simulink model "analisisDinamico2017"  (R2017a)
settings: Solver=VariableStepAuto  StartTime=0.0  StopTime=fin  FixedStep=0.001  RelTol=1e-3
values from neighbouring files (symbols this model uses):
  Aa1 = 1    [A_1_Obtencion_Modelo_Simbolico.m]    (also in modeloSimbolico.mat)
  Aa2 = Im2_cc*0.7    (= 2.59)    [A_1_Obtencion_Modelo_Simbolico.m]    (also in modeloSimbolico.mat)
  Aa3 = Im3_cc*0.6    (= 0.6)    [A_1_Obtencion_Modelo_Simbolico.m]    (also in modeloSimbolico.mat)
  Ab1 = 0.5    [A_1_Obtencion_Modelo_Simbolico.m]    (also in modeloSimbolico.mat)
  Ab2 = Aa2*0.8    (= 2.072)    [A_1_Obtencion_Modelo_Simbolico.m]    (also in modeloSimbolico.mat)
  Ab3 = Aa3*0.62    (= 0.372)    [A_1_Obtencion_Modelo_Simbolico.m]    (also in modeloSimbolico.mat)
  noise = 0.01    [A_1_Obtencion_Modelo_Simbolico.m]    (also in modeloSimbolico.mat)
  q2ini = -0.80020550259323    (= -0.800205502593)    [A_1_Obtencion_Modelo_Simbolico.m]    (also in modeloSimbolico.mat)
  q3ini = 0.202600802956157    (= 0.202600802956)    [A_1_Obtencion_Modelo_Simbolico.m]    (also in modeloSimbolico.mat)
  R1 = 50    [A_1_Obtencion_Modelo_Simbolico.m]    (also in A_2_Modelo_medidas_muestreado.m; A_2_Modelo_medidas_perfectas.m; modeloSimbolico.mat)
  R2 = 30    [A_1_Obtencion_Modelo_Simbolico.m]    (also in A_2_Modelo_medidas_muestreado.m; A_2_Modelo_medidas_perfectas.m; modeloSimbolico.mat)
  R3 = 15    [A_1_Obtencion_Modelo_Simbolico.m]    (also in A_2_Modelo_medidas_muestreado.m; A_2_Modelo_medidas_perfectas.m; modeloSimbolico.mat)
  Tau1 = 8    [A_1_Obtencion_Modelo_Simbolico.m]    (also in modeloSimbolico.mat)
  Tau2 = 15    [A_1_Obtencion_Modelo_Simbolico.m]    (also in modeloSimbolico.mat)
  Tau3 = 20    [A_1_Obtencion_Modelo_Simbolico.m]    (also in modeloSimbolico.mat)
  Ts = 0.001    [A_1_Obtencion_Modelo_Simbolico.m]    (also in modeloSimbolico.mat)
  wa1 = 1.3    [A_1_Obtencion_Modelo_Simbolico.m]    (also in modeloSimbolico.mat)
  wa2 = 3    [A_1_Obtencion_Modelo_Simbolico.m]    (also in modeloSimbolico.mat)
  wa3 = 5    [A_1_Obtencion_Modelo_Simbolico.m]    (also in modeloSimbolico.mat)
  wb1 = wa1*5    (= 6.5)    [A_1_Obtencion_Modelo_Simbolico.m]    (also in modeloSimbolico.mat)
  wb2 = wa2*3.5    (= 10.5)    [A_1_Obtencion_Modelo_Simbolico.m]    (also in modeloSimbolico.mat)
  wb3 = wa3*2.2    (= 11)    [A_1_Obtencion_Modelo_Simbolico.m]    (also in modeloSimbolico.mat)
undefined symbols (not defined in the file or in its folder): modeloIdeal, modeloReal
settings Model: Creator=Richa  LastModifiedBy=richard

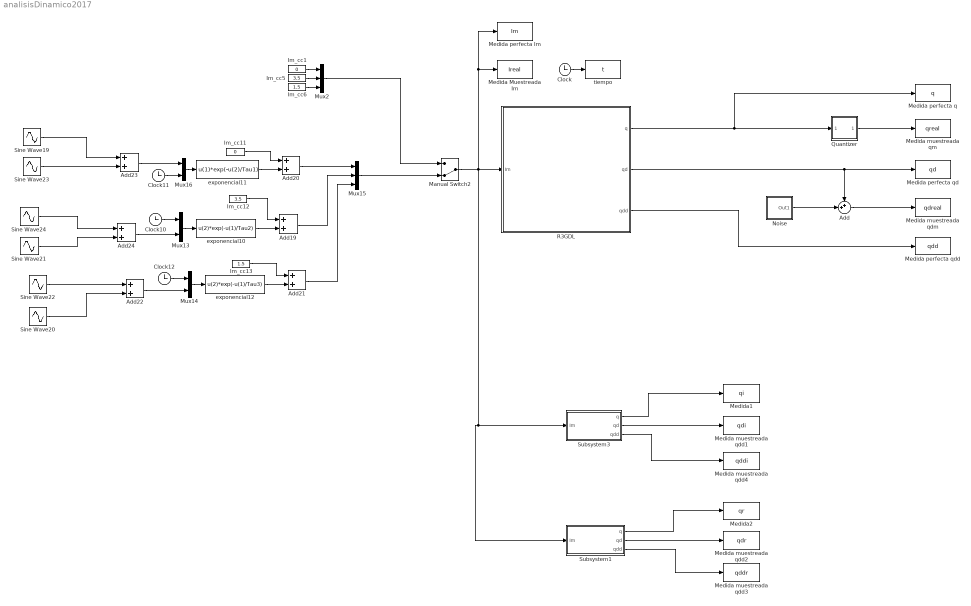
== system analisisDinamico2017 ==
  Add : Sum  Inputs=++|
  Add{19..24} (6 alike) : Sum
  Clock{,10..12} (4 alike) : Clock
  Im_cc1 : Constant  Value=0
  Im_cc11 : Constant  Value=0
  Im_cc12 : Constant  Value=3.5
  Im_cc13 : Constant  Value=1.5
  Im_cc5 : Constant  Value=3.5
  Im_cc6 : Constant  Value=1.5
  Manual Switch2 : ManualSwitch  CurrentSetting=0
  Medida Muestreada Im : ToWorkspace  VariableName=Ireal  SampleTime=Ts
  Medida muestreada qdd1 : ToWorkspace  VariableName=qdi  SampleTime=Ts
  Medida muestreada qdd2 : ToWorkspace  VariableName=qdr  SampleTime=Ts
  Medida muestreada qdd3 : ToWorkspace  VariableName=qddr  SampleTime=Ts
  Medida muestreada qdd4 : ToWorkspace  VariableName=qddi  SampleTime=Ts
  Medida muestreada qdm : ToWorkspace  VariableName=qdreal  SampleTime=Ts
  Medida muestreada qm : ToWorkspace  VariableName=qreal  SampleTime=Ts
  Medida perfecta Im : ToWorkspace  VariableName=Im  SampleTime=-1
  Medida perfecta q : ToWorkspace  VariableName=q  SampleTime=-1
  Medida perfecta qd : ToWorkspace  VariableName=qd  SampleTime=-1
  Medida perfecta qdd : ToWorkspace  VariableName=qdd  SampleTime=-1
  Medida1 : ToWorkspace  VariableName=qi  SampleTime=Ts
  Medida2 : ToWorkspace  VariableName=qr  SampleTime=Ts
  Mux13 : Mux  Inputs=2
  Mux14 : Mux  Inputs=2
  Mux15 : Mux  Inputs=3
  Mux16 : Mux  Inputs=2
  Mux2 : Mux  Inputs=3
  "Noise " : Subsystem
  "Quantizer " : Subsystem
  R3GDL : Subsystem  mask(Control y Programación de Robots (4 GIERM)){NGrupo=15, q1_ini=0, q2_ini=q2ini, q3_ini=q3ini, Bl_q1=off, Bl_q2=off, Bl_q3=off, AccionamientoDirecto=off}
      mask prompts: NGrupo "Nº de GRUPO"; q1_ini "q1 inicial  (rad)"; q2_ini "q2 inicial (rad)"; q3_ini "q3_inicial (rad)"; Bl_q1 "Bloqueo q1"; Bl_q2 "Bloqueo q2"; Bl_q3 "Bloqueo q3"; AccionamientoDirecto "Accionamiento directo"
      mask help: Robot de 3 grados de libertad RRR
      mask Display:
      | image(imread('R3GDL_RRR.JPG'));
      | port_label('output', 1, 'q');
      | port_label('output', 2, 'qd');
      | port_label('output', 3, 'qdd');
      | port_label('input', 1, 'Im')
  Sine Wave19 : Sin  Amplitude=Aa1  Frequency=wa1  SampleTime=0
  Sine Wave20 : Sin  Amplitude=Ab3  Frequency=wb3  SampleTime=0
  Sine Wave21 : Sin  Amplitude=Ab2  Frequency=wb2  SampleTime=0
  Sine Wave22 : Sin  Amplitude=Aa3  Frequency=wa3  SampleTime=0
  Sine Wave23 : Sin  Amplitude=Ab1  Frequency=wb1  SampleTime=0
  Sine Wave24 : Sin  Amplitude=Aa2  Frequency=wa2  SampleTime=0
  Subsystem1 : Subsystem
  Subsystem3 : Subsystem
  exponencial10 : Fcn  Expr=u(2)*exp(-u(1)/Tau2)
  exponencial11 : Fcn  Expr=u(1)*exp(-u(2)/Tau1)
  exponencial12 : Fcn  Expr=u(2)*exp(-u(1)/Tau3)
  tiempo : ToWorkspace  VariableName=t  SampleTime=Ts
  wires:
  "Quantizer "/1(Out1) -> Medida muestreada qm/1
  R3GDL/1(q) -> Medida perfecta q/1, "Quantizer "/1(In1)
  R3GDL/2(qd) -> Medida perfecta qd/1, Add/1
  "Noise "/1(Out1) -> Add/2
  Add/1 -> Medida muestreada qdm/1
  R3GDL/3(qdd) -> Medida perfecta qdd/1
  Manual Switch2/1 -> Medida perfecta Im/1, Medida Muestreada Im/1, Subsystem1/1(Im), Subsystem3/1(Im), R3GDL/1(Im)
  Clock/1 -> tiempo/1
  Add19/1 -> Mux15/2
  Im_cc12/1 -> Add19/1
  Clock10/1 -> Mux13/1
  Mux13/1 -> exponencial10/1
  exponencial10/1 -> Add19/2
  Add24/1 -> Mux13/2
  Sine Wave24/1 -> Add24/1
  Sine Wave21/1 -> Add24/2
  Add21/1 -> Mux15/3
  Mux14/1 -> exponencial12/1
  Clock12/1 -> Mux14/1
  Sine Wave20/1 -> Add22/2
  Add22/1 -> Mux14/2
  exponencial12/1 -> Add21/2
  Sine Wave22/1 -> Add22/1
  Im_cc13/1 -> Add21/1
  Im_cc11/1 -> Add20/1
  Clock11/1 -> Mux16/2
  Add23/1 -> Mux16/1
  Add20/1 -> Mux15/1
  Sine Wave23/1 -> Add23/2
  Mux16/1 -> exponencial11/1
  Sine Wave19/1 -> Add23/1
  exponencial11/1 -> Add20/2
  Mux2/1 -> Manual Switch2/1
  Im_cc1/1 -> Mux2/1
  Im_cc5/1 -> Mux2/2
  Im_cc6/1 -> Mux2/3
  Subsystem3/3(qdd) -> Medida muestreada qdd4/1
  Subsystem3/2(qd) -> Medida muestreada qdd1/1
  Subsystem3/1(q) -> Medida1/1
  Mux15/1 -> Manual Switch2/2
  Subsystem1/1(q) -> Medida2/1
  Subsystem1/2(qd) -> Medida muestreada qdd2/1
  Subsystem1/3(qdd) -> Medida muestreada qdd3/1

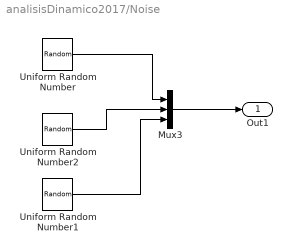
== system analisisDinamico2017/Noise  ==
  Mux3 : Mux  Inputs=3
  Uniform Random Number : UniformRandomNumber  Minimum=-(1500*2*pi/60)*(noise/R1)  Maximum=(1500*2*pi/60)*(noise/R1)  SampleTime=Ts*2
  Uniform Random Number1 : UniformRandomNumber  Minimum=-(1500*2*pi/60)*(noise/R3)  Maximum=(1500*2*pi/60)*(noise/R3)  SampleTime=Ts*2
  Uniform Random Number2 : UniformRandomNumber  Minimum=-(1500*2*pi/60)*(noise/R2)  Maximum=(1500*2*pi/60)*(noise/R2)  SampleTime=Ts*2
  Out1 : Outport
  wires:
  Uniform Random Number1/1 -> Mux3/3
  Uniform Random Number/1 -> Mux3/1
  Uniform Random Number2/1 -> Mux3/2
  Mux3/1 -> Out1/1

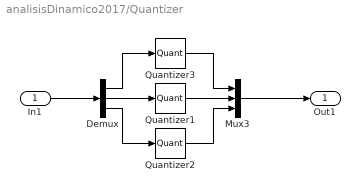
== system analisisDinamico2017/Quantizer  ==
  In1 : Inport
  Demux : Demux  Outputs=3
  Mux3 : Mux  Inputs=3
  Quantizer1 : Quantizer  QuantizationInterval=2*pi/1024/30
  Quantizer2 : Quantizer  QuantizationInterval=2*pi/1024/15
  Quantizer3 : Quantizer  QuantizationInterval=2*pi/1024/50
  Out1 : Outport
  wires:
  Demux/2 -> Quantizer1/1
  Mux3/1 -> Out1/1
  Quantizer1/1 -> Mux3/2
  Quantizer3/1 -> Mux3/1
  Quantizer2/1 -> Mux3/3
  In1/1 -> Demux/1
  Demux/3 -> Quantizer2/1
  Demux/1 -> Quantizer3/1

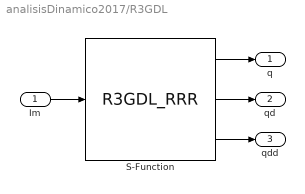
== system analisisDinamico2017/R3GDL ==
  Im : Inport
  S-Function : S-Function  FunctionName=R3GDL_RRR  Parameters=[q1_ini; q2_ini; q3_ini]; [Bl_q1; Bl_q2; Bl_q3]; AccionamientoDirecto; NGrupo  SFunctionDeploymentMode=off  EnableBusSupport=off
  q : Outport
  qd : Outport  Port=2
  qdd : Outport  Port=3
  wires:
  Im/1 -> S-Function/1
  S-Function/1 -> q/1
  S-Function/2 -> qd/1
  S-Function/3 -> qdd/1

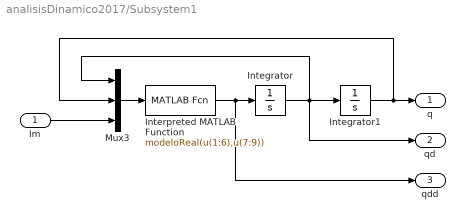
== system analisisDinamico2017/Subsystem1 ==
  Im : Inport
  Integrator : Integrator
  Integrator1 : Integrator  InitialCondition=[0 q2ini q3ini]
  Interpreted MATLAB Function : MATLABFcn  MATLABFcn=modeloReal(u(1:6),u(7:9))  OutputDimensions=3
  Mux3 : Mux  Inputs=3
  q : Outport
  qd : Outport  Port=2
  qdd : Outport  Port=3
  wires:
  Im/1 -> Mux3/3
  Integrator/1 -> Integrator1/1, Mux3/1, qd/1
  Interpreted MATLAB Function/1 -> qdd/1, Integrator/1
  Integrator1/1 -> q/1, Mux3/2
  Mux3/1 -> Interpreted MATLAB Function/1

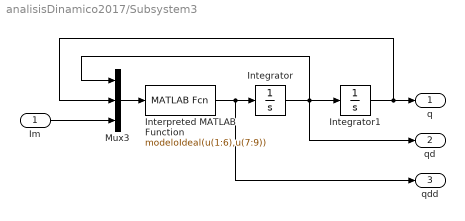
== system analisisDinamico2017/Subsystem3 ==
  Im : Inport
  Integrator : Integrator
  Integrator1 : Integrator  InitialCondition=[0 q2ini q3ini]
  Interpreted MATLAB Function : MATLABFcn  MATLABFcn=modeloIdeal(u(1:6),u(7:9))  OutputDimensions=3
  Mux3 : Mux  Inputs=3
  q : Outport
  qd : Outport  Port=2
  qdd : Outport  Port=3
  wires:
  Mux3/1 -> Interpreted MATLAB Function/1
  Integrator1/1 -> Mux3/2, q/1
  Interpreted MATLAB Function/1 -> Integrator/1, qdd/1
  Integrator/1 -> qd/1, Mux3/1, Integrator1/1
  Im/1 -> Mux3/3
